simulink model "IEEE34BARRAS"  (R2018a)
settings: Solver=ode4  StartTime=0.0  StopTime=48*T  FixedStep=Ts  RelTol=1e-3  EnableMultiTasking=on
InitFcn:
  | close
  | clc
  | clear
  | n=2^8;
  | f=60;
  | T=1/f;
  | Ts=1/(f*n);
  | NT=18;
  | set_param('IEEE34BARRAS/EMISOR-RECEPTOR/TCP_IP_RX1/ESCRITURA', 'Value','[0,0,0,0,0,0,0,0,0,0,0,0,0,0,0,0,0,0,0,0,0,0,0,0,0,0,0,0,0,0,0,0,0,0,0,0,0,0,0,0,0]')
  | set_param('IEEE34BARRAS/EMISOR-RECEPTOR/TCP_IP_RX1/RETARDO', 'Value','0')
  | run script_client_1_inicio1.m
undefined symbols (not defined in the file or in its folder): D1, Delta, DiscIntNeverNeededParam, Ip1
libraries: powerlib x313, simulink x15, libreria_medidores1 x3, libreria_comunicaciones_cliente1 x2
(part 5 of 5)

== system IEEE34BARRAS/RL4/RMS1/Hold derivative till next zero crossing1 ==
  note: Sample and Hold
  note: Silvano Casoria
      | Power System Simulation Laboratory
      | IREQ, Hydro-Quebc
  In : Inport
  S : Inport  Port=2
  Memory : Memory
  Switch : Switch  Threshold=0.5  SaturateOnIntegerOverflow=on  InputSameDT=on
  "   " : Outport  InitialOutput=0
  wires:
  Switch/1 -> "   "/1, Memory/1
  Memory/1 -> Switch/3
  In/1 -> Switch/1
  S/1 -> Switch/2

== system IEEE34BARRAS/RL4/RMS1/Hold derivative till next zero crossing2 ==
  note: Silvano Casoria
      | Power System Simulation Laboratory
      | IREQ, Hydro-Quebc
  note: Sample and Hold
  In : Inport
  S : Inport  Port=2
  Memory : Memory
  Switch : Switch  Threshold=0.5  SaturateOnIntegerOverflow=on  InputSameDT=on
  "   " : Outport  InitialOutput=0
  wires:
  S/1 -> Switch/2
  In/1 -> Switch/1
  Memory/1 -> Switch/3
  Switch/1 -> Memory/1, "   "/1

== system IEEE34BARRAS/RL5/RMS1/Hold derivative till next zero crossing ==
  note: Silvano Casoria
      | Power System Simulation Laboratory
      | IREQ, Hydro-Quebc
  note: Sample and Hold
  In : Inport
  S : Inport  Port=2
  Memory : Memory
  Switch : Switch  Threshold=0.5  SaturateOnIntegerOverflow=on  InputSameDT=on
  "   " : Outport  InitialOutput=0
  wires:
  S/1 -> Switch/2
  In/1 -> Switch/1
  Memory/1 -> Switch/3
  Switch/1 -> Memory/1, "   "/1

== system IEEE34BARRAS/RL5/RMS1/Hold derivative till next zero crossing1 ==
  note: Sample and Hold
  note: Silvano Casoria
      | Power System Simulation Laboratory
      | IREQ, Hydro-Quebc
  In : Inport
  S : Inport  Port=2
  Memory : Memory
  Switch : Switch  Threshold=0.5  SaturateOnIntegerOverflow=on  InputSameDT=on
  "   " : Outport  InitialOutput=0
  wires:
  Switch/1 -> "   "/1, Memory/1
  Memory/1 -> Switch/3
  In/1 -> Switch/1
  S/1 -> Switch/2

== system IEEE34BARRAS/RL5/RMS1/Hold derivative till next zero crossing2 ==
  note: Silvano Casoria
      | Power System Simulation Laboratory
      | IREQ, Hydro-Quebc
  note: Sample and Hold
  In : Inport
  S : Inport  Port=2
  Memory : Memory
  Switch : Switch  Threshold=0.5  SaturateOnIntegerOverflow=on  InputSameDT=on
  "   " : Outport  InitialOutput=0
  wires:
  S/1 -> Switch/2
  In/1 -> Switch/1
  Memory/1 -> Switch/3
  Switch/1 -> Memory/1, "   "/1
